simulink model "m_library"  (R2024b)
settings: Solver=FixedStepAuto  StartTime=0.0  StopTime=0.2  FixedStep=1e-4  RelTol=1e-4
undefined symbols (not defined in the file): DiscIntNeverNeededParam
settings Model: Creator=Jarvis  LastModifiedBy=32114

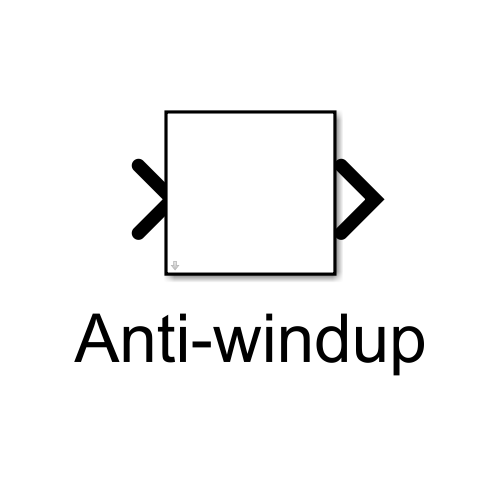
[thumbnail: Simulink's stored preview of the top-level diagram]
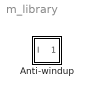
== system m_library ==
  Anti-windup : Subsystem  mask{Kp=0, Ki=0, Kb=0, Upper=0, Lower=0, Ts=-1}
      mask prompts: Kp "Proportion gain:"; Ki "Integration gain:"; Kb "Anti-saturation gain(alpha*ki/kp):"; Upper "Upper limit:"; Lower "Lower limit:"; Ts "Sampling time:"
      mask DialogControl ParameterGroupVar Prompt: 参数
      mask Display: %disp('Anti-windup')

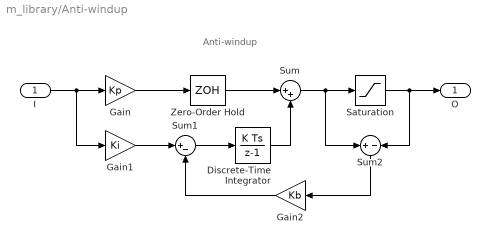
== system m_library/Anti-windup ==
  note: Anti-windup
  I : Inport
  Discrete-Time Integrator : DiscreteIntegrator  SampleTime=Ts  ICPrevOutput=DiscIntNeverNeededParam  ICPrevScaledInput=DiscIntNeverNeededParam
  Gain : Gain  Gain=Kp
  Gain1 : Gain  Gain=Ki
  Gain2 : Gain  Gain=Kb
  Saturation : Saturate  UpperLimit=Upper  LowerLimit=Lower
  Sum : Sum  Inputs=|++
  Sum1 : Sum  Inputs=|+-
  Sum2 : Sum  Inputs=+-
  Zero-Order Hold : ZeroOrderHold  SampleTime=Ts
  O : Outport
  wires:
  Sum/1 -> Sum2/1, Saturation/1
  Sum2/1 -> Gain2/1
  I/1 -> Gain1/1, Gain/1
  Saturation/1 -> O/1, Sum2/2
  Discrete-Time Integrator/1 -> Sum/2
  Sum1/1 -> Discrete-Time Integrator/1
  Gain/1 -> Zero-Order Hold/1
  Zero-Order Hold/1 -> Sum/1
  Gain1/1 -> Sum1/1
  Gain2/1 -> Sum1/2
